simulink model "Module 3"  (R2021b)
settings: Solver=FixedStepAuto  StartTime=0.0  StopTime=5  FixedStep=0.001  RelTol=1e-3
undefined symbols (not defined in the file or in its folder): magnitude
settings Model: Creator=Lenovo  LastModifiedBy=Lenovo

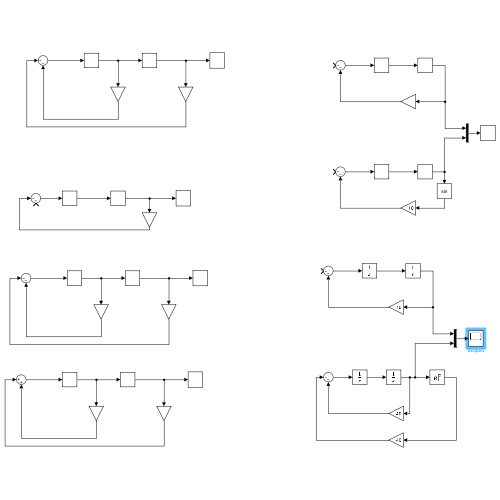
[thumbnail: Simulink's stored preview of the top-level diagram]
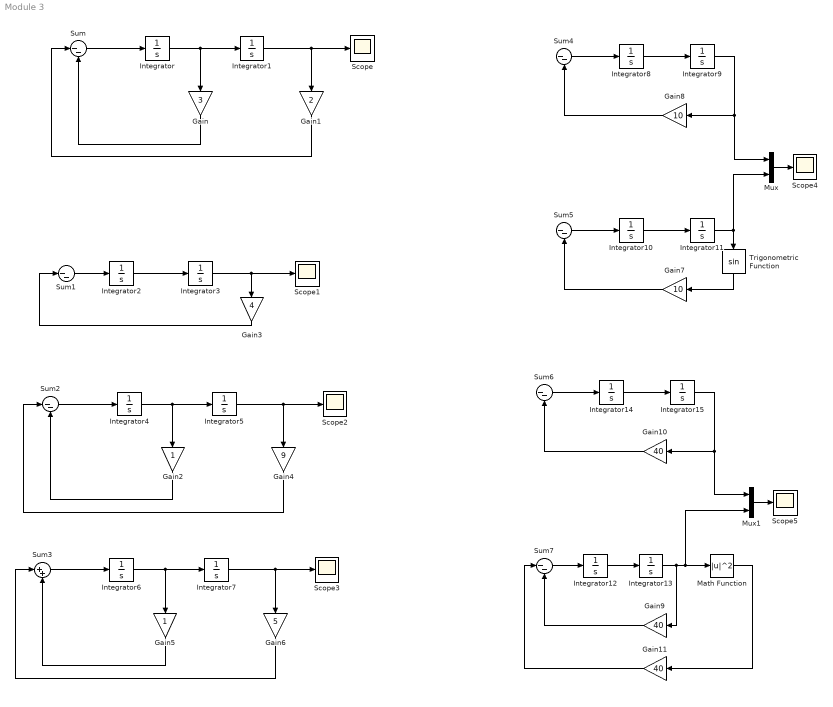
== system Module 3 ==
  Gain : Gain  Gain=3
  Gain1 : Gain  Gain=2
  Gain10 : Gain  Gain=40
  Gain11 : Gain  Gain=40
  Gain2 : Gain
  Gain3 : Gain  Gain=4
  Gain4 : Gain  Gain=9
  Gain5 : Gain
  Gain6 : Gain  Gain=5
  Gain7 : Gain  Gain=10
  Gain8 : Gain  Gain=10
  Gain9 : Gain  Gain=40
  Integrator : Integrator  InitialCondition=5
  Integrator1 : Integrator  InitialCondition=1
  Integrator{3..4,7..8,10,12,14} (7 alike) : Integrator
  Integrator{2,5..6,9,11} (5 alike) : Integrator  InitialCondition=0.1
  Integrator13 : Integrator  InitialCondition=0.3
  Integrator15 : Integrator  InitialCondition=0.3
  Math Function : Math  Operator=magnitude^2  SaturateOnIntegerOverflow=on
  Mux : Mux  Inputs=2
  Mux1 : Mux  Inputs=2
  Scope{,1..5} (6 alike) : Scope
  Sum{,1..2,4..7} (7 alike) : Sum  Inputs=|--
  Sum3 : Sum  Inputs=|++
  Trigonometric Function : Trigonometry
  wires:
  Sum/1 -> Integrator/1
  Integrator/1 -> Integrator1/1, Gain/1
  Integrator1/1 -> Gain1/1, Scope/1
  Gain/1 -> Sum/2
  Gain1/1 -> Sum/1
  Integrator2/1 -> Integrator3/1
  Gain3/1 -> Sum1/1
  Integrator3/1 -> Scope1/1, Gain3/1
  Sum1/1 -> Integrator2/1
  Gain2/1 -> Sum2/2
  Integrator4/1 -> Integrator5/1, Gain2/1
  Gain4/1 -> Sum2/1
  Integrator5/1 -> Gain4/1, Scope2/1
  Sum2/1 -> Integrator4/1
  Integrator7/1 -> Gain6/1, Scope3/1
  Sum3/1 -> Integrator6/1
  Gain5/1 -> Sum3/2
  Gain6/1 -> Sum3/1
  Integrator6/1 -> Integrator7/1, Gain5/1
  Integrator8/1 -> Integrator9/1
  Integrator9/1 -> Mux/1, Gain8/1
  Sum4/1 -> Integrator8/1
  Gain8/1 -> Sum4/2
  Mux/1 -> Scope4/1
  Sum5/1 -> Integrator10/1
  Integrator11/1 -> Mux/2, Trigonometric Function/1
  Integrator10/1 -> Integrator11/1
  Gain7/1 -> Sum5/2
  Trigonometric Function/1 -> Gain7/1
  Gain10/1 -> Sum6/2
  Integrator15/1 -> Mux1/1, Gain10/1
  Sum6/1 -> Integrator14/1
  Mux1/1 -> Scope5/1
  Integrator13/1 -> Math Function/1, Mux1/2, Gain9/1
  Sum7/1 -> Integrator12/1
  Integrator12/1 -> Integrator13/1
  Gain9/1 -> Sum7/2
  Integrator14/1 -> Integrator15/1
  Math Function/1 -> Gain11/1
  Gain11/1 -> Sum7/1
